simulink model "A421_example2"  (R2022b)
settings: Solver=VariableStepAuto  StartTime=0.0  StopTime=10.0  RelTol=1e-3
settings Model: Creator=willb  LastModifiedBy=willb

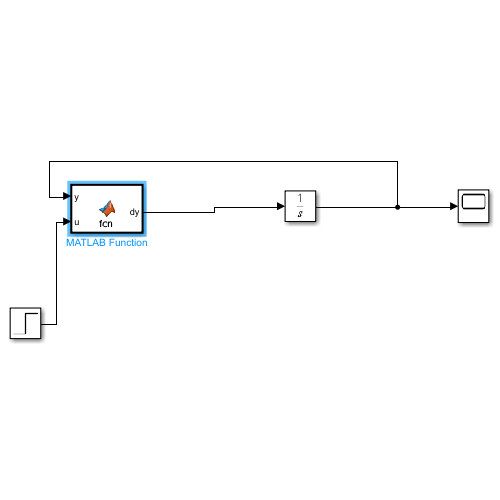
[thumbnail: Simulink's stored preview of the top-level diagram]
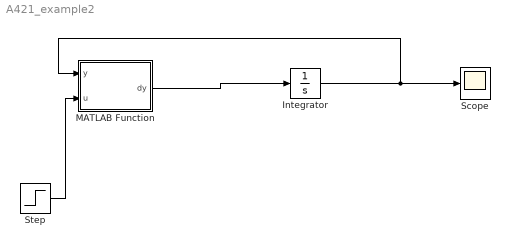
== system A421_example2 ==
  Integrator : Integrator
  MATLAB Function : MATLAB Function  TreatAsAtomicUnit=on
  Scope : Scope
  Step : Step  SampleTime=0
  wires:
  MATLAB Function/1(dy) -> Integrator/1
  Integrator/1 -> MATLAB Function/1(y), Scope/1
  Step/1 -> MATLAB Function/2(u)

== matlab function A421_example2/MATLAB Function ==
  data: y input; dy output; u input
function dy = fcn(y, u)

dy = [0;0];
z = 0.7;
w_n = 2;

dy(1) = y(2);
dy(2) = -2*z*w_n*y(1)-w_n^2*u;
